simulink model "lt2DPSK"  (R2016b)
settings: Solver=VariableStepAuto  StartTime=0.0  StopTime=1  RelTol=1e-3
libraries: commchan3 x1, dsparch4 x1, commrandsrc3 x1, commsink2 x1
settings Model: Creator=white  LastModifiedBy=white

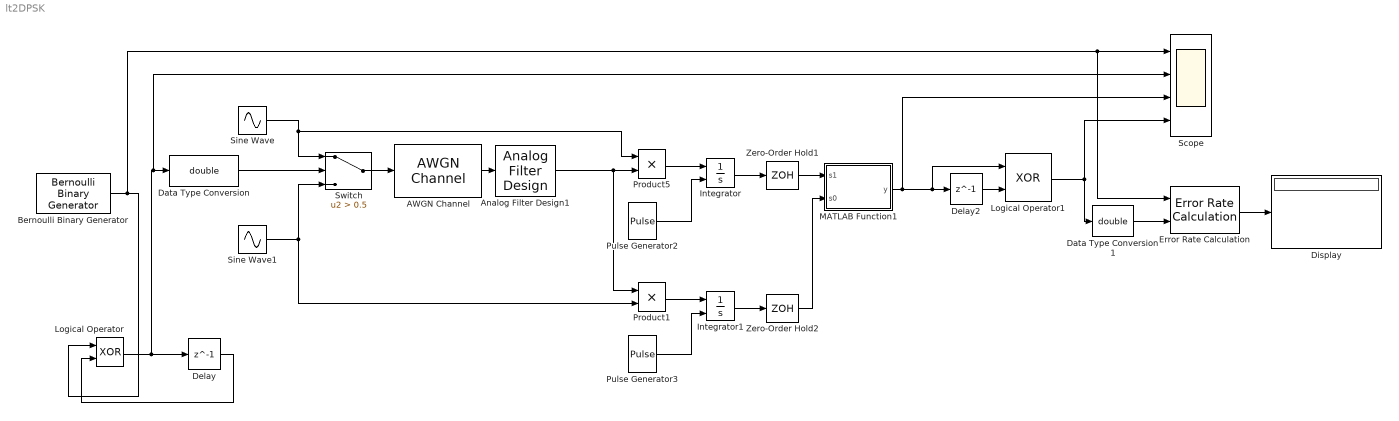
== system lt2DPSK ==
  AWGN Channel : commchan3/AWGN Channel  InputProcessing=Columns as channels (frame based)  seed=67  noiseMode=Variance from mask  EbNodB=10  EsNodB=10  SNRdB=10  bitsPerSym=800  Ps=1  Tsym=1  variance=0.01
  Analog Filter Design1 : dsparch4/Analog Filter Design  method=Butterworth  filttype=Bandpass  N=1  Wlo=2*24300*pi  Whi=2*25300*pi  Rp=2  Rs=40
  Bernoulli Binary Generator : commrandsrc3/Bernoulli Binary Generator  ProbabilityOfZero=0.5  SeedSource=Auto  Seed=0  SampleTime=0.00125  SamplesPerFrame=1  OutputDataType=double  SimulateUsing=Interpreted execution
  Data Type Conversion : DataTypeConversion  OutDataTypeStr=double
  Data Type Conversion1 : DataTypeConversion  OutDataTypeStr=double
  Delay : Delay  DelayLength=1  InitialCondition=0  SampleTime=1/800
  Delay2 : Delay  DelayLength=1  InitialCondition=0  SampleTime=1/800
  Display : Display
  Error Rate Calculation : commsink2/Error Rate Calculation  N=1  st_delay=0  cp_mode=Entire frame  subframe=[]  PMode=Port  WsName=ErrorVec  RsMode2=off  stop=off  numErr=100  maxBits=1e6
  Integrator : Integrator  ExternalReset=rising
  Integrator1 : Integrator  ExternalReset=rising
  Logical Operator : Logic  Operator=XOR  AllPortsSameDT=off  OutDataTypeStr=boolean
  Logical Operator1 : Logic  Operator=XOR  AllPortsSameDT=off  OutDataTypeStr=boolean
  MATLAB Function1 : MATLAB Function  TreatAsAtomicUnit=on
  Product1 : Product
  Product5 : Product
  Pulse Generator2 : DiscretePulseGenerator  PulseType=Time based  Period=1/800  PulseWidth=5  PhaseDelay=1/1600
  Pulse Generator3 : DiscretePulseGenerator  PulseType=Time based  Period=1/800  PulseWidth=5  PhaseDelay=1/1600
  Scope : Scope  NumInputPorts=4
  Sine Wave : Sin  Frequency=2*24800*pi  SampleTime=0
  Sine Wave1 : Sin  Frequency=2*pi*24800  Phase=pi  SampleTime=0
  Switch : Switch  Criteria=u2 > Threshold  Threshold=0.5
  Zero-Order Hold1 : ZeroOrderHold  SampleTime=1/800
  Zero-Order Hold2 : ZeroOrderHold  SampleTime=1/800
  wires:
  Logical Operator/1 -> Scope/2, Data Type Conversion/1, Delay/1
  Delay/1 -> Logical Operator/2
  Data Type Conversion/1 -> Switch/2
  Sine Wave1/1 -> Switch/3, Product1/2
  Switch/1 -> AWGN Channel/1
  AWGN Channel/1 -> Analog Filter Design1/1
  Integrator/1 -> Zero-Order Hold1/1
  Zero-Order Hold1/1 -> MATLAB Function1/1(s1)
  Delay2/1 -> Logical Operator1/2
  Product5/1 -> Integrator/1
  Pulse Generator2/1 -> Integrator/2
  MATLAB Function1/1(y) -> Scope/3, Logical Operator1/1, Delay2/1
  Integrator1/1 -> Zero-Order Hold2/1
  Analog Filter Design1/1 -> Product1/1, Product5/2
  Product1/1 -> Integrator1/1
  Pulse Generator3/1 -> Integrator1/2
  Sine Wave/1 -> Product5/1, Switch/1
  Zero-Order Hold2/1 -> MATLAB Function1/2(s0)
  Logical Operator1/1 -> Data Type Conversion1/1, Scope/4
  Error Rate Calculation/1 -> Display/1
  Bernoulli Binary Generator/1 -> Scope/1, Error Rate Calculation/1, Logical Operator/1
  Data Type Conversion1/1 -> Error Rate Calculation/2

== matlab function lt2DPSK/MATLAB Function1 ==
  data: s1 input; y output; s0 input
function y = fcn(s1,s0)
if(s1>=s0)
    u=1
else
    u=0
end
y = u;
